simulink model "Junctions5"  (Simulink 5.0)
settings: Solver=ode45  StartTime=0.0  StopTime=10.0  RelTol=1e-3
settings Model: Creator=scaife  LastModifiedBy=scaife  ExtModeAutoUpdateStatusClock=off

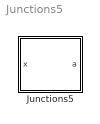
== system Junctions5 ==
  Junctions5 : Stateflow chart

== stateflow chart Junctions5 ==
  state A/
    ex: a+=10000
  state B/
    ex: a=0
  A -> (junction 5) : [x%%3==0]{a+=1}
  A -> (junction 5) : [x%%3==1]{a+=10}
  (junction 5) -> (junction 6) : [x>=2]{a+=100}
  (junction 6) -> B : [x>=4]{a+=1000}
  (default) -> A
  data: x input int32; a output double
